simulink model "lab3_1ed902"  (R2019b)
settings: Solver=FixedStepDiscrete  StartTime=0.0  StopTime=inf  FixedStep=0.006  RelTol=1e-3  EnableMultiTasking=on
undefined symbols (not defined in the file): DiscIntNeverNeededParam
libraries: simulink x3, MinSegLibrary_M1V4 x2, RASPlib x1, arduinolib x1
settings Model: SimulationMode=external  ExtModeTrigDuration=2  Creator=mapeac  LastModifiedBy=sb224sc
settings DataIOCC: ReturnWorkspaceOutputs=off
settings OptimizationCC: EnhancedBackFolding=on  PassReuseOutputArgsThreshold=0  MaxStackSize=64  OptimizeBlockOrder=speed  DifferentSizesBufferReuse=on  OptimizationCustomize=off
settings DebuggingCC: ParameterTunabilityLossMsg=error  ArithmeticOperatorsInVariantConditions=warning
settings HardwareCC: ProdBitPerInt=16  ProdBitPerPointer=16  ProdBitPerSizeT=16  ProdBitPerPtrDiffT=16  ProdLargestAtomicFloat=None  ProdWordSize=8  ProdHWDeviceType=Atmel->AVR  UseEmbeddedCoderFeatures=off  UseSimulinkCoderFeatures=off
settings SFSimCC: SimUseLocalCustomCode=off  MATLABDynamicMemAlloc=off  CustomCodeUndefinedFunction=UseInterfaceOnly
settings RTWCC: SystemTargetFile=ert.tlc  HardwareBoard=Arduino Mega 2560  TLCOptions=-aInlineSetEventsForThisBaseRateFcn=TLC_FALSE -aSuppressMultiTaskScheduler=TLC_FALSE -aRateBasedStepFcn=1  TemplateMakefile=ert_default_tmf  GenerateReport=on  RTWUseLocalCustomCode=off  Toolchain=Arduino AVR  BuildConfiguration=Faster Runs  LaunchReport=on
settings CodeAppCC: ForceParamTrailComments=on  OperatorAnnotations=on  MangleLength=10
settings ERTTargetCC: ERTCustomFileBanners=off  SupportContinuousTime=on  SupportNonInlinedSFcns=on  RemoveResetFunc=off  SupportVariableSizeSignals=on  ModelStepFunctionPrototypeControlCompliant=off

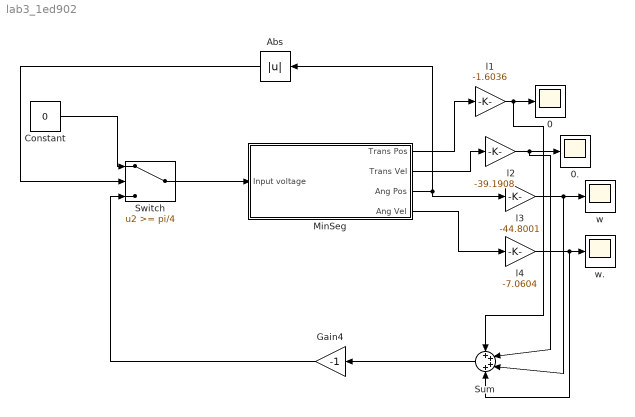
== system lab3_1ed902 ==
  0 : Scope
  0. : Scope
  Abs : Abs
  Constant : Constant  Value=0
  Gain4 : Gain  Gain=-1
  MinSeg : Subsystem
  Sum : Sum  Inputs=4
  Switch : Switch  Threshold=pi/4
  l1 : Gain  Gain=-1.6036
  l2 : Gain  Gain=-39.1908
  l3 : Gain  Gain=-44.8001
  l4 : Gain  Gain=-7.0604
  w : Scope
  w. : Scope
  wires:
  Abs/1 -> Switch/2
  MinSeg/3(Ang Pos) -> Abs/1, l3/1
  Switch/1 -> MinSeg/1(Input voltage)
  Constant/1 -> Switch/1
  MinSeg/1(Trans Pos) -> l1/1
  l1/1 -> Sum/1, 0/1
  l4/1 -> Sum/4, w./1
  MinSeg/4(Ang Vel) -> l4/1
  l3/1 -> Sum/3, w/1
  l2/1 -> Sum/2, 0./1
  MinSeg/2(Trans Vel) -> l2/1
  Sum/1 -> Gain4/1
  Gain4/1 -> Switch/3

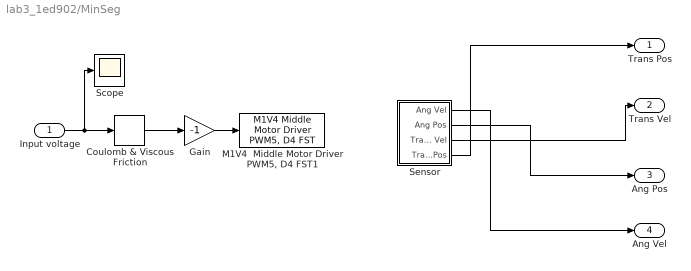
== system lab3_1ed902/MinSeg ==
  Input voltage : Inport
  Coulomb & Viscous Friction : simulink/Discontinuities/Coulomb & Viscous Friction  offset=0  gain=1
      settings: SourceProductName=Simulink
  Gain : Gain  Gain=-1
  "M1V4  Middle Motor Driver PWM5, D4 FST1" : MinSegLibrary_M1V4/M1V4  Middle Motor Driver PWM5, D4 FST  Vsupply=3.25
      settings: SourceProductName=Rensselaer Arduino Support Package
  Scope : Scope
  Sensor : Subsystem
  Trans Pos : Outport  VectorParamsAs1DForOutWhenUnconnected=off
  Trans Vel : Outport  Port=2  VectorParamsAs1DForOutWhenUnconnected=off
  Ang Pos : Outport  Port=3  VectorParamsAs1DForOutWhenUnconnected=off
  Ang Vel : Outport  Port=4  VectorParamsAs1DForOutWhenUnconnected=off
  wires:
  Sensor/3(Trans Vel) -> Trans Vel/1
  Sensor/4(Trans Pos) -> Trans Pos/1
  Sensor/2(Ang Pos) -> Ang Pos/1
  Sensor/1(Ang Vel) -> Ang Vel/1
  Gain/1 -> "M1V4  Middle Motor Driver PWM5, D4 FST1"/1
  Input voltage/1 -> Scope/1, Coulomb & Viscous Friction/1
  Coulomb & Viscous Friction/1 -> Gain/1

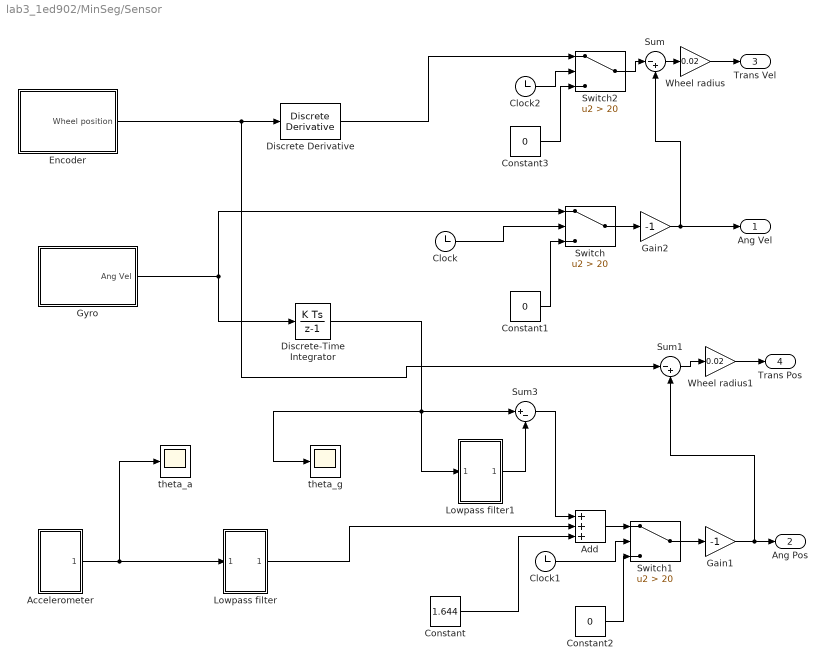
== system lab3_1ed902/MinSeg/Sensor ==
  Accelerometer : Subsystem
  Add : Sum  Inputs=+++
  Clock : Clock
  Clock1 : Clock
  Clock2 : Clock
  Constant : Constant  Value=1.644
  Constant1 : Constant  Value=0
  Constant2 : Constant  Value=0
  Constant3 : Constant  Value=0
  Discrete Derivative : simulink/Discrete/Discrete Derivative  gainval=1.0  ICPrevScaledInput=0.0  OutMin=[]  OutMax=[]  OutDataType=fixdt(1, 16)  OutScaling=2^-10  DoSatur=off
  Discrete-Time Integrator : DiscreteIntegrator  SampleTime=-1  ICPrevOutput=DiscIntNeverNeededParam  ICPrevScaledInput=DiscIntNeverNeededParam
  Encoder : Subsystem
  Gain1 : Gain  Gain=-1
  Gain2 : Gain  Gain=-1
  Gyro : Subsystem
  Lowpass filter : Subsystem
  Lowpass filter1 : Subsystem
  Sum : Sum  Inputs=|-+
  Sum1 : Sum  Inputs=|-+
  Sum3 : Sum  Inputs=|+-
  Switch : Switch  Criteria=u2 > Threshold  Threshold=20
  Switch1 : Switch  Criteria=u2 > Threshold  Threshold=20
  Switch2 : Switch  Criteria=u2 > Threshold  Threshold=20
  Wheel radius : Gain  Gain=0.02
  Wheel radius1 : Gain  Gain=0.02
  theta_a : Scope
  theta_g : Scope
  Ang Vel : Outport  VectorParamsAs1DForOutWhenUnconnected=off
  Ang Pos : Outport  Port=2  VectorParamsAs1DForOutWhenUnconnected=off
  Trans Vel : Outport  Port=3  VectorParamsAs1DForOutWhenUnconnected=off
  Trans Pos : Outport  Port=4  VectorParamsAs1DForOutWhenUnconnected=off
  wires:
  Gyro/1(Ang Vel) -> Switch/1, Discrete-Time Integrator/1
  Discrete-Time Integrator/1 -> Lowpass filter1/1(In1), Sum3/1, theta_g/1
  Lowpass filter1/1(Out1) -> Sum3/2
  Add/1 -> Switch1/1
  Accelerometer/1(Ang Pos) -> theta_a/1, Lowpass filter/1(In1)
  Constant/1 -> Add/3
  Lowpass filter/1(Out1) -> Add/2
  Sum3/1 -> Add/1
  Switch/1 -> Gain2/1
  Constant1/1 -> Switch/3
  Clock/1 -> Switch/2
  Clock1/1 -> Switch1/2
  Constant2/1 -> Switch1/3
  Constant3/1 -> Switch2/3
  Clock2/1 -> Switch2/2
  Discrete Derivative/1 -> Switch2/1
  Gain1/1 -> Sum1/2, Ang Pos/1
  Switch1/1 -> Gain1/1
  Gain2/1 -> Sum/2, Ang Vel/1
  Switch2/1 -> Sum/1
  Sum/1 -> Wheel radius/1
  Wheel radius/1 -> Trans Vel/1
  Sum1/1 -> Wheel radius1/1
  Wheel radius1/1 -> Trans Pos/1
  Encoder/1(Wheel position) -> Sum1/1, Discrete Derivative/1

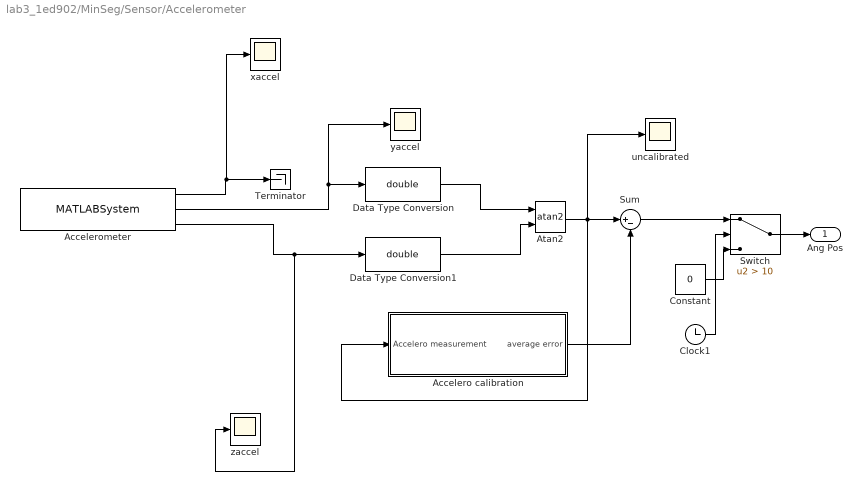
== system lab3_1ed902/MinSeg/Sensor/Accelerometer ==
  Accelero calibration : Subsystem
  Accelerometer : MATLABSystem  System=soMPU6050Accel  SimulateUsing=Code generation
      mask Type: soMPU6050Accel
      mask Display:
      | disp('soMPU6050Accel');
      | port_label('output',1,'xaccel');
      | port_label('output',2,'yaccel');
      | port_label('output',3,'zaccel');
  Atan2 : Trigonometry  Operator=atan2
  Clock1 : Clock
  Constant : Constant  Value=0
  Data Type Conversion : DataTypeConversion  OutDataTypeStr=double
  Data Type Conversion1 : DataTypeConversion  OutDataTypeStr=double
  Sum : Sum  Inputs=|+-
  Switch : Switch  Criteria=u2 > Threshold  Threshold=10
  Terminator : Terminator
  uncalibrated : Scope
  xaccel : Scope
  yaccel : Scope
  zaccel : Scope
  Ang Pos : Outport  VectorParamsAs1DForOutWhenUnconnected=off
  wires:
  Data Type Conversion1/1 -> Atan2/2
  Accelerometer/2 -> Data Type Conversion/1, yaccel/1
  Atan2/1 -> uncalibrated/1, Sum/1, Accelero calibration/1(Accelero measurement)
  Accelerometer/3 -> zaccel/1, Data Type Conversion1/1
  Data Type Conversion/1 -> Atan2/1
  Accelerometer/1 -> xaccel/1, Terminator/1
  Accelero calibration/1(average error) -> Sum/2
  Sum/1 -> Switch/1
  Constant/1 -> Switch/3
  Clock1/1 -> Switch/2
  Switch/1 -> Ang Pos/1

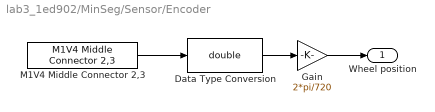
== system lab3_1ed902/MinSeg/Sensor/Encoder ==
  Data Type Conversion : DataTypeConversion  OutDataTypeStr=double
  Gain : Gain  Gain=2*pi/720
  M1V4 Middle Connector 2,3 : MinSegLibrary_M1V4/M1V4 Middle Connector 2,3  Encoder=0  PinA=3  PinB=2
      settings: SourceProductName=Rensselaer Arduino Support Package
  Wheel position : Outport  VectorParamsAs1DForOutWhenUnconnected=off
  wires:
  M1V4 Middle Connector 2,3/1 -> Data Type Conversion/1
  Data Type Conversion/1 -> Gain/1
  Gain/1 -> Wheel position/1

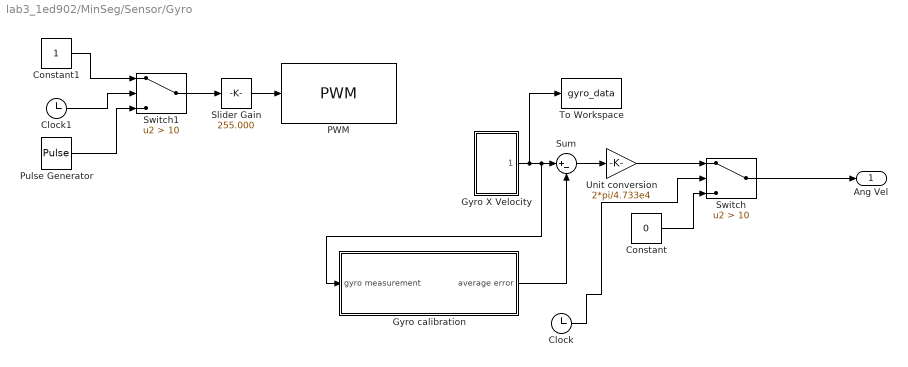
== system lab3_1ed902/MinSeg/Sensor/Gyro ==
  Clock : Clock
  Clock1 : Clock
  Constant : Constant  Value=0
  Constant1 : Constant
  Gyro X Velocity : Subsystem
  Gyro calibration : Subsystem
  PWM : arduinolib/PWM  pinNumber=13  EnableInputFrequency=off  InitialFrequency=2000  InitialDutyCycle=0  NotificationType=None  blockPlatform=arduino
  Pulse Generator : DiscretePulseGenerator  PulseType=Time based  Period=0.6  PulseWidth=50
  Slider Gain : simulink/Math Operations/Slider Gain  gain=255.000  low=0  high=255
  Sum : Sum  Inputs=|+-
  Switch : Switch  Criteria=u2 > Threshold  Threshold=10
  Switch1 : Switch  Criteria=u2 > Threshold  Threshold=10
  To Workspace : ToWorkspace  VariableName=gyro_data  SampleTime=-1
  Unit conversion : Gain  Gain=2*pi/4.733e4
  Ang Vel : Outport  VectorParamsAs1DForOutWhenUnconnected=off
  wires:
  Gyro calibration/1(average error) -> Sum/2
  Clock/1 -> Switch/2
  Gyro X Velocity/1(gyro out) -> Gyro calibration/1(gyro measurement), Sum/1, To Workspace/1
  Unit conversion/1 -> Switch/1
  Switch/1 -> Ang Vel/1
  Constant/1 -> Switch/3
  Sum/1 -> Unit conversion/1
  Pulse Generator/1 -> Switch1/3
  Slider Gain/1 -> PWM/1
  Constant1/1 -> Switch1/1
  Clock1/1 -> Switch1/2
  Switch1/1 -> Slider Gain/1

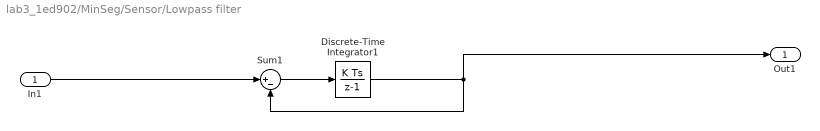
== system lab3_1ed902/MinSeg/Sensor/Lowpass filter ==
  In1 : Inport
  Discrete-Time Integrator1 : DiscreteIntegrator  gainval=3  SampleTime=-1  ICPrevOutput=DiscIntNeverNeededParam  ICPrevScaledInput=DiscIntNeverNeededParam
  Sum1 : Sum  Inputs=|+-
  Out1 : Outport  VectorParamsAs1DForOutWhenUnconnected=off
  wires:
  Discrete-Time Integrator1/1 -> Out1/1, Sum1/2
  Sum1/1 -> Discrete-Time Integrator1/1
  In1/1 -> Sum1/1

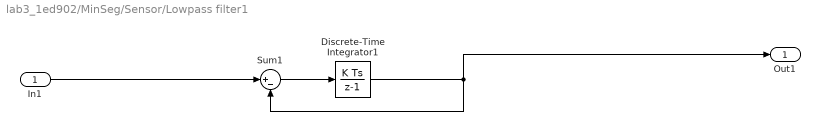
== system lab3_1ed902/MinSeg/Sensor/Lowpass filter1 ==
  In1 : Inport
  Discrete-Time Integrator1 : DiscreteIntegrator  gainval=3  SampleTime=-1  ICPrevOutput=DiscIntNeverNeededParam  ICPrevScaledInput=DiscIntNeverNeededParam
  Sum1 : Sum  Inputs=|+-
  Out1 : Outport  VectorParamsAs1DForOutWhenUnconnected=off
  wires:
  Discrete-Time Integrator1/1 -> Out1/1, Sum1/2
  Sum1/1 -> Discrete-Time Integrator1/1
  In1/1 -> Sum1/1

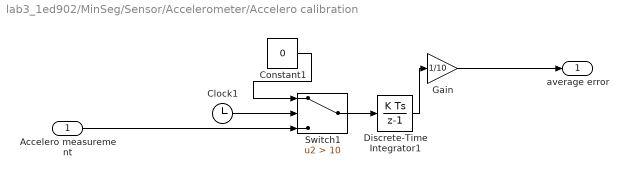
== system lab3_1ed902/MinSeg/Sensor/Accelerometer/Accelero calibration ==
  Accelero measurement : Inport
  Clock1 : Clock
  Constant1 : Constant  Value=0
  Discrete-Time Integrator1 : DiscreteIntegrator  SampleTime=-1  ICPrevOutput=DiscIntNeverNeededParam  ICPrevScaledInput=DiscIntNeverNeededParam
  Gain : Gain  Gain=1/10
  Switch1 : Switch  Criteria=u2 > Threshold  Threshold=10
  average error : Outport  VectorParamsAs1DForOutWhenUnconnected=off
  wires:
  Switch1/1 -> Discrete-Time Integrator1/1
  Constant1/1 -> Switch1/1
  Clock1/1 -> Switch1/2
  Accelero measurement/1 -> Switch1/3
  Discrete-Time Integrator1/1 -> Gain/1
  Gain/1 -> average error/1

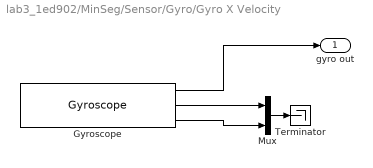
== system lab3_1ed902/MinSeg/Sensor/Gyro/Gyro X Velocity ==
  Gyroscope : RASPlib/Gyroscope  DLPFmode=5
      settings: SourceProductName=Rensselaer Arduino Support Package
  Mux : Mux  Inputs=2
  Terminator : Terminator
  gyro out : Outport  VectorParamsAs1DForOutWhenUnconnected=off
  wires:
  Gyroscope/1 -> gyro out/1
  Gyroscope/2 -> Mux/1
  Mux/1 -> Terminator/1
  Gyroscope/3 -> Mux/2

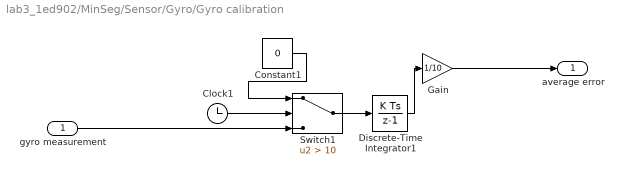
== system lab3_1ed902/MinSeg/Sensor/Gyro/Gyro calibration ==
  gyro measurement : Inport
  Clock1 : Clock
  Constant1 : Constant  Value=0
  Discrete-Time Integrator1 : DiscreteIntegrator  SampleTime=-1  ICPrevOutput=DiscIntNeverNeededParam  ICPrevScaledInput=DiscIntNeverNeededParam
  Gain : Gain  Gain=1/10
  Switch1 : Switch  Criteria=u2 > Threshold  Threshold=10
  average error : Outport  VectorParamsAs1DForOutWhenUnconnected=off
  wires:
  Switch1/1 -> Discrete-Time Integrator1/1
  Constant1/1 -> Switch1/1
  Clock1/1 -> Switch1/2
  gyro measurement/1 -> Switch1/3
  Discrete-Time Integrator1/1 -> Gain/1
  Gain/1 -> average error/1
